simulink model "Nalanchira_RMU_"  (R2025b)
settings: Solver=VariableStepAuto  StartTime=0.0  StopTime=0.81  RelTol=1e-3
libraries: spsThreePhaseFaultLib x12, spsThreePhaseBreakerLib x8, spsThreePhasePISectionLineLib x6, spsThreePhaseVIMeasurementLib x4, spsThreePhaseSourceLib x2, spsThreePhaseParallelRLCLoadLib x2, spsThreePhaseTransformerTwoWindingsLib x2, sps_lib x1
settings Model: Creator=sheya  LastModifiedBy=sheya
settings DataIOCC: SaveOutput=off  SaveTime=off

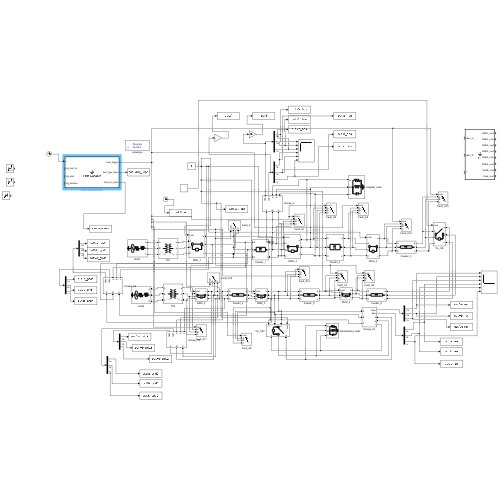
[thumbnail: Simulink's stored preview of the top-level diagram]
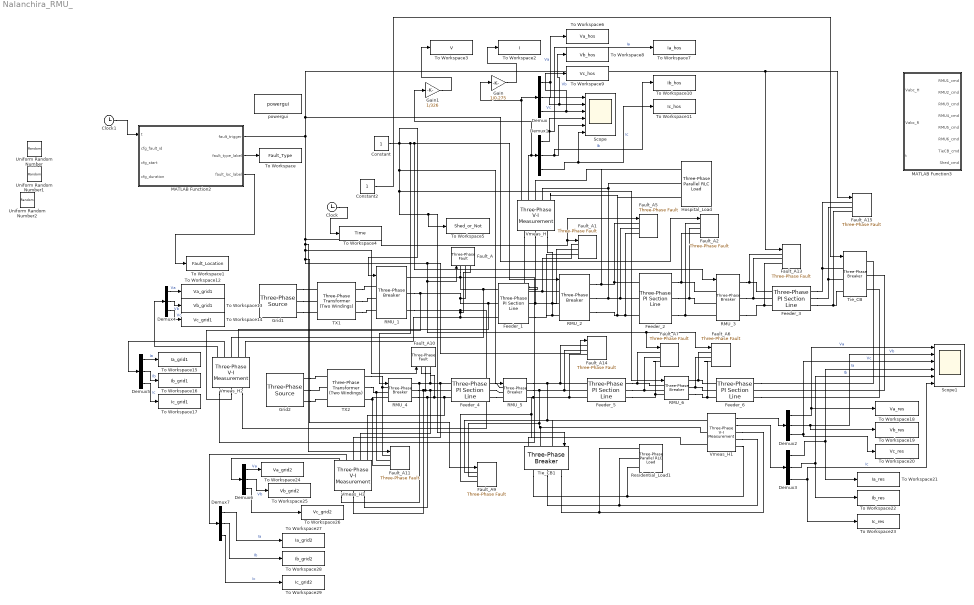
== system Nalanchira_RMU_ ==
  Clock : Clock
  Clock1 : Clock
  Constant : Constant
  Constant2 : Constant
  Demux{,1..7} (8 alike) : Demux  Outputs=3
  Fault_A : spsThreePhaseFaultLib/Three-Phase Fault  InitialStates=0  FaultA=on  FaultB=on  FaultC=on  GroundFault=on  SwitchTimes="[0.2  0.5]"  External=on  SwitchStatus=NaN  FaultResistance=0.001  GroundResistance=0.01  SnubberResistance=1e6  SnubberCapacitance=inf  Measurements=None
  Fault_A1 : spsThreePhaseFaultLib/Three-Phase Fault  InitialStates=0  FaultA=off  FaultB=on  FaultC=on  GroundFault=on  SwitchTimes="[0.2  0.5]"  External=on  SwitchStatus=NaN  FaultResistance=0.001  GroundResistance=0.01  SnubberResistance=1e6  SnubberCapacitance=inf  Measurements=None
  Fault_A10 : spsThreePhaseFaultLib/Three-Phase Fault  InitialStates=0  FaultA=on  FaultB=on  FaultC=on  GroundFault=off  SwitchTimes="[0.2  0.5]"  External=on  SwitchStatus=NaN  FaultResistance=0.001  GroundResistance=0.01  SnubberResistance=1e6  SnubberCapacitance=inf  Measurements=None
  Fault_A11 : spsThreePhaseFaultLib/Three-Phase Fault  InitialStates=0  FaultA=off  FaultB=off  FaultC=on  GroundFault=on  SwitchTimes="[0.2  0.5]"  External=on  SwitchStatus=NaN  FaultResistance=0.001  GroundResistance=0.01  SnubberResistance=1e6  SnubberCapacitance=inf  Measurements=None
  Fault_A13 : spsThreePhaseFaultLib/Three-Phase Fault  InitialStates=0  FaultA=on  FaultB=on  FaultC=on  GroundFault=on  SwitchTimes="[0.2  0.5]"  External=on  SwitchStatus=NaN  FaultResistance=0.001  GroundResistance=0.01  SnubberResistance=1e6  SnubberCapacitance=inf  Measurements=None
  Fault_A14 : spsThreePhaseFaultLib/Three-Phase Fault  InitialStates=0  FaultA=off  FaultB=on  FaultC=off  GroundFault=on  SwitchTimes="[0.2  0.5]"  External=on  SwitchStatus=NaN  FaultResistance=0.001  GroundResistance=0.01  SnubberResistance=1e6  SnubberCapacitance=inf  Measurements=None
  Fault_A15 : spsThreePhaseFaultLib/Three-Phase Fault  InitialStates=0  FaultA=on  FaultB=on  FaultC=on  GroundFault=on  SwitchTimes="[0.2  0.5]"  External=on  SwitchStatus=NaN  FaultResistance=0.001  GroundResistance=0.01  SnubberResistance=1e6  SnubberCapacitance=inf  Measurements=None
  Fault_A2 : spsThreePhaseFaultLib/Three-Phase Fault  InitialStates=0  FaultA=on  FaultB=off  FaultC=on  GroundFault=on  SwitchTimes="[0.2  0.5]"  External=on  SwitchStatus=NaN  FaultResistance=0.001  GroundResistance=0.01  SnubberResistance=1e6  SnubberCapacitance=inf  Measurements=None
  Fault_A5 : spsThreePhaseFaultLib/Three-Phase Fault  InitialStates=0  FaultA=off  FaultB=on  FaultC=on  GroundFault=off  SwitchTimes="[0.2  0.5]"  External=on  SwitchStatus=NaN  FaultResistance=0.001  GroundResistance=0.01  SnubberResistance=1e6  SnubberCapacitance=inf  Measurements=None
  Fault_A6 : spsThreePhaseFaultLib/Three-Phase Fault  InitialStates=0  FaultA=on  FaultB=off  FaultC=on  GroundFault=on  SwitchTimes="[0.2  0.5]"  External=on  SwitchStatus=NaN  FaultResistance=0.001  GroundResistance=0.01  SnubberResistance=1e6  SnubberCapacitance=inf  Measurements=None
  Fault_A7 : spsThreePhaseFaultLib/Three-Phase Fault  InitialStates=0  FaultA=on  FaultB=on  FaultC=on  GroundFault=off  SwitchTimes="[0.2  0.5]"  External=on  SwitchStatus=NaN  FaultResistance=0.001  GroundResistance=0.01  SnubberResistance=1e6  SnubberCapacitance=inf  Measurements=None
  Fault_A9 : spsThreePhaseFaultLib/Three-Phase Fault  InitialStates=0  FaultA=on  FaultB=on  FaultC=off  GroundFault=off  SwitchTimes="[0.2  0.5]"  External=on  SwitchStatus=NaN  FaultResistance=0.001  GroundResistance=0.01  SnubberResistance=1e6  SnubberCapacitance=inf  Measurements=None
  Feeder_{1..6} (6 alike) : spsThreePhasePISectionLineLib/Three-Phase PI Section Line  LConnTagsString=a|b|c  RConnTagsString=A|B|C  Length=100  Frequency=60  Resistances=[ 0.01273 0.3864]  Inductances="[ 0.9337e-3  4.1264e-3]"  Capacitances=[12.74e-9 7.751e-9]
  Gain : Gain  Gain=1/0.275
  Gain1 : Gain  Gain=1/326
  Grid1 : spsThreePhaseSourceLib/Three-Phase Source  InternalConnection=Yg  VoltagePhases=off  Voltage=11000  PhaseAngle=0  Voltage_phases=[25e3 25e3 25e3]/sqrt(3)  PhaseAngles_phases=[0 -120 +120]  Frequency=50  NonIdealSource=on  SpecifyImpedance=off  Resistance=0.8929  Inductance=16.58e-3  ShortCircuitLevel=100e6  BaseVoltage=25e3  XRratio=7  BusType=swing  Pref=10e3  Qref=0  Prefabc=[10e3, 10e3, 10e3]  Qrefabc=[0, 0, 0]  Qmin=-inf  Qmax=inf
  Grid2 : spsThreePhaseSourceLib/Three-Phase Source  InternalConnection=Yg  VoltagePhases=off  Voltage=11000  PhaseAngle=0  Voltage_phases=[25e3 25e3 25e3]/sqrt(3)  PhaseAngles_phases=[0 -120 +120]  Frequency=50  NonIdealSource=on  SpecifyImpedance=off  Resistance=0.8929  Inductance=16.58e-3  ShortCircuitLevel=100e6  BaseVoltage=25e3  XRratio=7  BusType=swing  Pref=10e3  Qref=0  Prefabc=[10e3, 10e3, 10e3]  Qrefabc=[0, 0, 0]  Qmin=-inf  Qmax=inf
  Hospital_Load : spsThreePhaseParallelRLCLoadLib/Three-Phase Parallel RLC Load  LConnTagsString=A|B|C  Configuration=Y (grounded)  NominalVoltage=11000  Vabc=[1e3 1e3 1e3]  Vabcp=[1e3 1e3 1e3]  NominalFrequency=60  UnbalancedPower=off  ActivePower=10e3  InductivePower=100  CapacitivePower=100  Pabc=[10e3 9e3 11e3]  QLabc=[100 90 110]  QCabc=[100 90 110]  Pabcp=[10e3 9e3 11e3]  QLabcp=[100 90 110]  QCabcp=[100 90 110]  Measurements=None  LoadType=constant Z
  MATLAB Function2 : MATLAB Function  TreatAsAtomicUnit=on
  MATLAB Function3 : MATLAB Function  TreatAsAtomicUnit=on
  RMU_{1..6} (6 alike) : spsThreePhaseBreakerLib/Three-Phase Breaker  InitialState=closed  SwitchA=on  SwitchB=on  SwitchC=on  SwitchTimes="[1/60  5/60]"  External=on  BreakerResistance=0.01  SnubberResistance=1e6  SnubberCapacitance=inf  Measurements=None
  Residential_Load1 : spsThreePhaseParallelRLCLoadLib/Three-Phase Parallel RLC Load  LConnTagsString=A|B|C  Configuration=Y (grounded)  NominalVoltage=11000  Vabc=[1e3 1e3 1e3]  Vabcp=[1e3 1e3 1e3]  NominalFrequency=60  UnbalancedPower=off  ActivePower=10e3  InductivePower=100  CapacitivePower=100  Pabc=[10e3 9e3 11e3]  QLabc=[100 90 110]  QCabc=[100 90 110]  Pabcp=[10e3 9e3 11e3]  QLabcp=[100 90 110]  QCabcp=[100 90 110]  Measurements=None  LoadType=constant Z
  Scope : Scope  NumInputPorts=6
      settings: ActiveDisplayYMinimum=-420.61136129921823  ActiveDisplayYMaximum=420.62339836741489  YLabel=Voltage (Volts)
  Scope1 : Scope  NumInputPorts=6
      settings: ActiveDisplayYMinimum=-420.51879516691815  ActiveDisplayYMaximum=420.5442993232071  YLabel=Voltage (Volts)
  TX1 : spsThreePhaseTransformerTwoWindingsLib/Three-Phase Transformer (Two Windings)  Winding1Connection=Yg  Winding2Connection=Yg  CoreType=Three single-phase transformers  SetSaturation=off  Hysteresis=off  DataFile='hysteresis'  SetInitialFlux=off  Measurements=None  UNITS=pu  NominalPower=[ 500e3 , 60 ]  Winding1=[ 11000 , 0.002 , 0.08 ]  Winding2=[ 400 , 0.002 , 0.08 ]  Rm=500  Lm=500  L0=0.5  Saturation=[ 0,0 ; 0.0024,1.2 ; 1.0,1.52 ]  InitialFluxes=[ 0.8 , -0.8 , 0.7 ]  BreakLoop=off  DiscreteSolver=Trapezoidal iterative  DataType=off  TransfoNumber=1
  TX2 : spsThreePhaseTransformerTwoWindingsLib/Three-Phase Transformer (Two Windings)  Winding1Connection=Yg  Winding2Connection=Yg  CoreType=Three single-phase transformers  SetSaturation=off  Hysteresis=off  DataFile='hysteresis'  SetInitialFlux=off  Measurements=None  UNITS=pu  NominalPower=[ 500e3 , 60 ]  Winding1=[ 11000 , 0.002 , 0.08 ]  Winding2=[ 400 , 0.002 , 0.08 ]  Rm=500  Lm=500  L0=0.5  Saturation=[ 0,0 ; 0.0024,1.2 ; 1.0,1.52 ]  InitialFluxes=[ 0.8 , -0.8 , 0.7 ]  BreakLoop=off  DiscreteSolver=Trapezoidal iterative  DataType=off  TransfoNumber=1
  Tie_CB : spsThreePhaseBreakerLib/Three-Phase Breaker  InitialState=open  SwitchA=on  SwitchB=on  SwitchC=on  SwitchTimes="[1/60  5/60]"  External=on  BreakerResistance=0.01  SnubberResistance=1e6  SnubberCapacitance=inf  Measurements=None
  Tie_CB1 : spsThreePhaseBreakerLib/Three-Phase Breaker  InitialState=open  SwitchA=on  SwitchB=on  SwitchC=on  SwitchTimes="[1/60  5/60]"  External=on  BreakerResistance=0.01  SnubberResistance=1e6  SnubberCapacitance=inf  Measurements=None
  To Workspace : ToWorkspace  VariableName=Fault_Type  SampleTime=-1
  To Workspace1 : ToWorkspace  VariableName=Fault_Location  SampleTime=-1
  To Workspace10 : ToWorkspace  VariableName=Ib_hos  SampleTime=-1
  To Workspace11 : ToWorkspace  VariableName=Ic_hos  SampleTime=-1
  To Workspace12 : ToWorkspace  VariableName=Va_grid1  SampleTime=-1
  To Workspace13 : ToWorkspace  VariableName=Vb_grid1  SampleTime=-1
  To Workspace14 : ToWorkspace  VariableName=Vc_grid1  SampleTime=-1
  To Workspace15 : ToWorkspace  VariableName=Ia_grid1  SampleTime=-1
  To Workspace16 : ToWorkspace  VariableName=Ib_grid1  SampleTime=-1
  To Workspace17 : ToWorkspace  VariableName=Ic_grid1  SampleTime=-1
  To Workspace18 : ToWorkspace  VariableName=Va_res  SampleTime=-1
  To Workspace19 : ToWorkspace  VariableName=Vb_res  SampleTime=-1
  To Workspace2 : ToWorkspace  VariableName=I  SampleTime=-1
  To Workspace20 : ToWorkspace  VariableName=Vc_res  SampleTime=-1
  To Workspace21 : ToWorkspace  VariableName=Ia_res  SampleTime=-1
  To Workspace22 : ToWorkspace  VariableName=Ib_res  SampleTime=-1
  To Workspace23 : ToWorkspace  VariableName=Ic_res  SampleTime=-1
  To Workspace24 : ToWorkspace  VariableName=Va_grid2  SampleTime=-1
  To Workspace25 : ToWorkspace  VariableName=Vb_grid2  SampleTime=-1
  To Workspace26 : ToWorkspace  VariableName=Vc_grid2  SampleTime=-1
  To Workspace27 : ToWorkspace  VariableName=Ia_grid2  SampleTime=-1
  To Workspace28 : ToWorkspace  VariableName=Ib_grid2  SampleTime=-1
  To Workspace29 : ToWorkspace  VariableName=Ic_grid2  SampleTime=-1
  To Workspace3 : ToWorkspace  VariableName=V  SampleTime=-1
  To Workspace4 : ToWorkspace  VariableName=Time  SampleTime=-1
  To Workspace5 : ToWorkspace  VariableName=Shed_or_Not  SampleTime=-1
  To Workspace6 : ToWorkspace  VariableName=Va_hos  SampleTime=-1
  To Workspace7 : ToWorkspace  VariableName=Ia_hos  SampleTime=-1
  To Workspace8 : ToWorkspace  VariableName=Vb_hos  SampleTime=-1
  To Workspace9 : ToWorkspace  VariableName=Vc_hos  SampleTime=-1
  Uniform Random Number : UniformRandomNumber  Minimum=1  Maximum=16  SampleTime=1
  Uniform Random Number1 : UniformRandomNumber  Minimum=0.2  Maximum=0.6  SampleTime=1
  Uniform Random Number2 : UniformRandomNumber  Minimum=0.55  Maximum=0.6  SampleTime=1
  Vmeas_H{,1..3} (4 alike) : spsThreePhaseVIMeasurementLib/Three-Phase V-I Measurement  VoltageMeasurement=phase-to-ground  SetLabelV=off  LabelV=Vabc  Vpu=off  VpuLL=off  CurrentMeasurement=yes  SetLabelI=off  LabelI=Iabc  Ipu=off  Pbase=100e6  Vbase=500e3  OutputType=Complex  PhasorSimulation=off  PSBequivalent=0
  powergui : sps_lib/powergui  Priority=1  SimulationMode=Discrete  SampleTime=50e-6  frequency=60  Iterations=50  frequencyindice=0  Pbase=100e6  ErrMax=1e-4  UnitsV=kV  UnitsW=MW  buscounter=0  FunctionMessages=off  echomessages=off  EnableUseOfTLC=off  CurrentSourceSwitches=off  DisableSnubberDevices=off  DisableRonSwitches=off  DisableVfSwitches=off  DisplayEquations=off  AutomaticDiscreteSolvers=off  SolverType=Tustin/Backward Euler (TBE)  Interpol=off  ExternalGateDelay=off  methode=off  Ts=100  x0status=blocks  SPID=on  SwTol=0  HookPort=off  NonlinearTolerance=1e-4  nMaxIteration=100  ContinueOnMaxIteration=off  RestoreLinks=warning  ResistiveCurrentMeasurement=off  Frange=[0:2:500]  Ylog=off  Xlog=on  ShowGrid=off  save=off  variable=ZData  structure=0  ZoomFFT=off  StartTime=0.0  cycles=1  DisplayStyle=1  fundamental=60  FreqAxis=off  MaxFrequency=1000  frequencyindicesteady=1  RmsSteady=1  display=off
  wires:
  Clock/1 -> To Workspace4/1
  Constant/1 -> RMU_5/1, RMU_6/1, To Workspace5/1, Tie_CB1/1, RMU_4/1, RMU_3/1, RMU_2/1, RMU_1/1
  Vmeas_H/2 -> Gain1/1, Demux1/1
  Demux/1 -> To Workspace6/1, Scope/1  "Va"
  Demux2/1 -> To Workspace18/1, Scope1/1  "Va"
  Demux3/2 -> To Workspace22/1, Scope1/5  "Ib"
  Vmeas_H1/1 -> Demux2/1
  Demux2/2 -> To Workspace19/1, Scope1/2  "Vb"
  Vmeas_H1/2 -> Demux3/1
  Demux2/3 -> To Workspace20/1, Scope1/3  "Vc"
  Demux1/2 -> To Workspace10/1, Scope/5  "Ib"
  Demux3/3 -> To Workspace23/1, Scope1/6  "Ic"
  Demux/3 -> To Workspace9/1, Scope/3  "Vc"
  Demux1/1 -> To Workspace7/1, Scope/4  "Ia"
  Vmeas_H/1 -> Gain/1, Demux/1
  Demux/2 -> To Workspace8/1, Scope/2  "Vb"
  Demux1/3 -> To Workspace11/1, Scope/6  "Ic"
  MATLAB Function2/2(fault_type_label) -> To Workspace/1
  MATLAB Function2/3(fault_loc_label) -> To Workspace1/1
  MATLAB Function2/1(fault_trigger) -> Fault_A6/1, Fault_A7/1, Fault_A/1, Fault_A14/1, Fault_A9/1, Fault_A10/1, Fault_A11/1, Fault_A5/1, Fault_A1/1, Fault_A15/1, Fault_A13/1, Fault_A2/1
  Gain1/1 -> To Workspace3/1
  Gain/1 -> To Workspace2/1
  Vmeas_H2/1 -> Demux4/1
  Vmeas_H2/2 -> Demux5/1
  Demux4/1 -> To Workspace12/1  "Va"
  Demux4/2 -> To Workspace13/1  "Vb"
  Demux4/3 -> To Workspace14/1  "Vc"
  Demux5/1 -> To Workspace15/1  "Ia"
  Demux5/2 -> To Workspace16/1  "Ib"
  Demux5/3 -> To Workspace17/1  "Ic"
  Demux3/1 -> To Workspace21/1, Scope1/4  "Ia"
  Vmeas_H3/1 -> Demux6/1
  Vmeas_H3/2 -> Demux7/1
  Demux6/1 -> To Workspace24/1  "Va"
  Demux6/2 -> To Workspace25/1  "Vb"
  Demux6/3 -> To Workspace26/1
  Demux7/1 -> To Workspace27/1  "Ia"
  Demux7/2 -> To Workspace28/1  "Ib"
  Demux7/3 -> To Workspace29/1  "Ic"
  Constant2/1 -> Tie_CB/1
  Clock1/1 -> MATLAB Function2/1(t)
  connections:
  Residential_Load1/LConn3 -- Tie_CB1/RConn3 -- Vmeas_H1/RConn3
  Fault_A9/LConn1 -- Tie_CB1/LConn1 -- Vmeas_H1/LConn1 -- RMU_5/RConn1 -- Fault_A14/LConn1 -- Feeder_5/LConn1
  Vmeas_H1/RConn1 -- Tie_CB1/RConn1 -- Residential_Load1/LConn1
  Vmeas_H1/RConn2 -- Tie_CB1/RConn2 -- Residential_Load1/LConn2
  Vmeas_H/RConn2 -- Fault_A5/LConn2 -- Feeder_2/LConn2 -- RMU_2/RConn2 -- Hospital_Load/LConn2
  Vmeas_H1/LConn2 -- RMU_5/RConn2 -- Fault_A14/LConn2 -- Feeder_5/LConn2 -- Fault_A9/LConn2 -- Tie_CB1/LConn2
  Feeder_1/RConn1 -- Vmeas_H/LConn1 -- Fault_A1/LConn1 -- RMU_2/LConn1
  RMU_2/RConn1 -- Hospital_Load/LConn1 -- Vmeas_H/RConn1 -- Fault_A5/LConn1 -- Feeder_2/LConn1
  Fault_A9/LConn3 -- Tie_CB1/LConn3 -- Vmeas_H1/LConn3 -- RMU_5/RConn3 -- Fault_A14/LConn3 -- Feeder_5/LConn3
  RMU_2/RConn3 -- Hospital_Load/LConn3 -- Vmeas_H/RConn3 -- Fault_A5/LConn3 -- Feeder_2/LConn3
  Feeder_1/RConn2 -- Fault_A1/LConn2 -- RMU_2/LConn2 -- Vmeas_H/LConn2
  RMU_2/LConn3 -- Fault_A1/LConn3 -- Feeder_1/RConn3 -- Vmeas_H/LConn3
  RMU_4/RConn1 -- Fault_A10/LConn1 -- Vmeas_H3/RConn1 -- Feeder_4/LConn1 -- Vmeas_H3/LConn1
  Feeder_4/RConn3 -- RMU_5/LConn3
  Feeder_5/RConn3 -- Fault_A7/LConn3 -- RMU_6/LConn3
  Feeder_4/RConn1 -- RMU_5/LConn1
  Feeder_3/RConn2 -- Fault_A15/LConn2 -- Tie_CB/LConn2
  Feeder_3/RConn1 -- Fault_A15/LConn1 -- Tie_CB/LConn1
  Grid2/RConn1 -- TX2/LConn1
  TX1/RConn2 -- RMU_1/LConn2
  TX1/RConn1 -- RMU_1/LConn1
  TX2/RConn2 -- Fault_A11/LConn2 -- RMU_4/LConn2
  TX1/RConn3 -- RMU_1/LConn3
  RMU_1/RConn3 -- Vmeas_H2/LConn3 -- Fault_A/LConn3 -- Feeder_1/LConn3 -- Vmeas_H2/RConn3
  TX2/RConn1 -- RMU_4/LConn1 -- Fault_A11/LConn1
  Feeder_2/RConn1 -- Fault_A2/LConn3 -- RMU_3/LConn1
  RMU_3/RConn1 -- Fault_A13/LConn1 -- Feeder_3/LConn1
  Feeder_6/RConn1 -- Tie_CB/RConn1
  Feeder_1/LConn1 -- Vmeas_H2/RConn1 -- RMU_1/RConn1 -- Vmeas_H2/LConn1 -- Fault_A/LConn1
  Feeder_6/RConn3 -- Tie_CB/RConn3
  RMU_6/RConn1 -- Fault_A6/LConn1 -- Feeder_6/LConn1
  TX2/RConn3 -- Fault_A11/LConn3 -- RMU_4/LConn3
  RMU_1/RConn2 -- Vmeas_H2/LConn2 -- Fault_A/LConn2 -- Vmeas_H2/RConn2 -- Feeder_1/LConn2
  Feeder_2/RConn3 -- RMU_3/LConn3 -- Fault_A2/LConn1
  RMU_6/RConn3 -- Fault_A6/LConn3 -- Feeder_6/LConn3
  Tie_CB/RConn2 -- Feeder_6/RConn2
  Grid1/RConn3 -- TX1/LConn3
  RMU_3/RConn2 -- Fault_A13/LConn2 -- Feeder_3/LConn2
  RMU_3/RConn3 -- Fault_A13/LConn3 -- Feeder_3/LConn3
  RMU_6/RConn2 -- Feeder_6/LConn2 -- Fault_A6/LConn2
  Feeder_2/RConn2 -- Fault_A2/LConn2 -- RMU_3/LConn2
  RMU_4/RConn3 -- Vmeas_H3/LConn3 -- Fault_A10/LConn3 -- Vmeas_H3/RConn3 -- Feeder_4/LConn3
  Feeder_3/RConn3 -- Fault_A15/LConn3 -- Tie_CB/LConn3
  Grid1/RConn1 -- TX1/LConn1
  Feeder_5/RConn2 -- Fault_A7/LConn2 -- RMU_6/LConn2
  RMU_4/RConn2 -- Vmeas_H3/LConn2 -- Feeder_4/LConn2 -- Vmeas_H3/RConn2 -- Fault_A10/LConn2
  Feeder_5/RConn1 -- Fault_A7/LConn1 -- RMU_6/LConn1
  Feeder_4/RConn2 -- RMU_5/LConn2
  Grid2/RConn3 -- TX2/LConn3
  Grid1/RConn2 -- TX1/LConn2
  Grid2/RConn2 -- TX2/LConn2

== matlab function Nalanchira_RMU_/MATLAB Function2 ==
  data: fault_trigger output; fault_type_label output; fault_loc_label output; t input; cfg_fault_id input; cfg_start input; cfg_duration input
function [fault_trigger, fault_type_label, fault_loc_label] = Fault_Manager(t, cfg_fault_id, cfg_start, cfg_duration)
    
    % 1. Static Mapping
    temp_map = [101, 101, 102, 102, 103, 104, 104, 105, 106, 107, 108, 109, 110, 111, 112];
    
    % 2. Safety Check (Prevents the "Index exceeds dimensions" error)
    if isempty(cfg_fault_id) || cfg_fault_id < 1 || cfg_fault_id > 15
        fault_trigger = 0;
        fault_type_label = 0;
        fault_loc_label = 0;
        return;
    end
    
    % 3. Logic Execution
    fault_type_label = double(cfg_fault_id); 
    fault_loc_label  = double(temp_map(cfg_fault_id));
    
    fault_trigger = 0;
    % Trigger only during the window passed from the script
    if t >= cfg_start && t <= (cfg_start + cfg_duration)
        fault_trigger = 1;
    end
end

== matlab function Nalanchira_RMU_/MATLAB Function3 ==
  data: Vabc_H input; RMU1_cmd output; Vabc_R input; RMU2_cmd output; RMU3_cmd output; RMU4_cmd output; RMU5_cmd output; RMU6_cmd output; TieCB_cmd output; Shed_cmd output; t input
function [RMU1_cmd, RMU2_cmd, RMU3_cmd, RMU4_cmd, RMU5_cmd, RMU6_cmd, TieCB_cmd, Shed_cmd] = fcn(Vabc_H, Vabc_R, t)
    
    % --- Step 1: Define Thresholds ---
   % Inside your MATLAB Function Block
V_nominal = 1.0; % Your observed peak from Workspace
V_min = 0.85; % Set threshold at 85% of nominal

    
    % Monitor the Hospital side voltage magnitude
    % Using max(abs()) is a quick way to check for a drop in any phase
  V_mag_H = mean(abs(Vabc_H)); 
    
    % --- Step 2: Normal Operation State ---
    % All RMUs are closed to allow normal flow
    RMU1_cmd = 1; 
    RMU2_cmd = 1;
    RMU3_cmd = 1;
    RMU4_cmd = 1;
    RMU5_cmd = 1;
    RMU6_cmd = 1;
    
    % Tie-Breaker is OPEN normally (0)
    TieCB_cmd = 0;
    
    % Load Shedding is OFF normally (0 = Load Connected)
    Shed_cmd = 0;

    % --- Step 3: Self-Healing Logic (Fault near Hospital) ---
    % We wait until t > 0.05 to avoid transient startup spikes
    if V_mag_H < V_min && t > 0.05
        
        % 1. Isolate the Hospital from the faulted Grid
        RMU1_cmd = 0;   
        
        % 2. Close the Tie-Breaker to bring power from Grid 1
        TieCB_cmd = 1;  
        
        % 3. Perform Load Shedding on Residential side 
        % This prevents Grid 1 from tripping due to the sudden combined load
        Shed_cmd = 1;   
        
        % Note: RMU2-RMU6 remain 1 to maintain the new power path
    end
end
